simulink model "SWC_HALOUT_type"  (R2021b)
settings: Solver=FixedStepDiscrete  StartTime=0.0  StopTime=10.0  FixedStep=0.005  RelTol=1e-3
values from neighbouring files (symbols this model uses):
  DTC_10020B = Simulink.Parameter    [DTC_Constant_Definition.m]
  DTC_10020C = Simulink.Parameter    [DTC_Constant_Definition.m]
  DTC_10020D = Simulink.Parameter    [DTC_Constant_Definition.m]
  DTC_10020E = Simulink.Parameter    [DTC_Constant_Definition.m]
  DTC_100210 = Simulink.Parameter    [DTC_Constant_Definition.m]
  DTC_100211 = Simulink.Parameter    [DTC_Constant_Definition.m]
  DTC_100212 = Simulink.Parameter    [DTC_Constant_Definition.m]
  DTC_100213 = Simulink.Parameter    [DTC_Constant_Definition.m]
  DTC_100214 = Simulink.Parameter    [DTC_Constant_Definition.m]
  DTC_100215 = Simulink.Parameter    [DTC_Constant_Definition.m]
  DTC_100216 = Simulink.Parameter    [DTC_Constant_Definition.m]
  DTC_100217 = Simulink.Parameter    [DTC_Constant_Definition.m]
  DTC_100218 = Simulink.Parameter    [DTC_Constant_Definition.m]
  DTC_100219 = Simulink.Parameter    [DTC_Constant_Definition.m]
  DTC_10021A = Simulink.Parameter    [DTC_Constant_Definition.m]
  DTC_10021B = Simulink.Parameter    [DTC_Constant_Definition.m]
  DTC_10021C = Simulink.Parameter    [DTC_Constant_Definition.m]
  DTC_10021D = Simulink.Parameter    [DTC_Constant_Definition.m]
  DTC_10021E = Simulink.Parameter    [DTC_Constant_Definition.m]
  DTC_100220 = Simulink.Parameter    [DTC_Constant_Definition.m]
  DTC_100221 = Simulink.Parameter    [DTC_Constant_Definition.m]
  DTC_100223 = Simulink.Parameter    [DTC_Constant_Definition.m]
  DTC_100224 = Simulink.Parameter    [DTC_Constant_Definition.m]
  DTC_100225 = Simulink.Parameter    [DTC_Constant_Definition.m]
  DTC_100226 = Simulink.Parameter    [DTC_Constant_Definition.m]
  DTC_100227 = Simulink.Parameter    [DTC_Constant_Definition.m]
  DTC_100242 = Simulink.Parameter    [DTC_Constant_Definition.m]
  DTC_100243 = Simulink.Parameter    [DTC_Constant_Definition.m]
  DTC_100244 = Simulink.Parameter    [DTC_Constant_Definition.m]
  DTC_100247 = Simulink.Parameter    [DTC_Constant_Definition.m]
  DTC_100248 = Simulink.Parameter    [DTC_Constant_Definition.m]
  DTC_100249 = Simulink.Parameter    [DTC_Constant_Definition.m]
  DTC_100250 = Simulink.Parameter    [DTC_Constant_Definition.m]
  DTC_100251 = Simulink.Parameter    [DTC_Constant_Definition.m]
  DTC_100252 = Simulink.Parameter    [DTC_Constant_Definition.m]
  DTC_100A10 = Simulink.Parameter    [DTC_Constant_Definition.m]
  DTC_100A12 = Simulink.Parameter    [DTC_Constant_Definition.m]
  DTC_100A16 = Simulink.Parameter    [DTC_Constant_Definition.m]
  DTC_100A17 = Simulink.Parameter    [DTC_Constant_Definition.m]
  DTC_100A18 = Simulink.Parameter    [DTC_Constant_Definition.m]
  DTC_100A19 = Simulink.Parameter    [DTC_Constant_Definition.m]
  DTC_500B01 = Simulink.Parameter    [DTC_Constant_Definition.m]
  DTC_500B02 = Simulink.Parameter    [DTC_Constant_Definition.m]
  DTC_500B03 = Simulink.Parameter    [DTC_Constant_Definition.m]
  DTC_500B04 = Simulink.Parameter    [DTC_Constant_Definition.m]
  DTC_500B05 = Simulink.Parameter    [DTC_Constant_Definition.m]
  DTC_500B06 = Simulink.Parameter    [DTC_Constant_Definition.m]
  DTC_500B07 = Simulink.Parameter    [DTC_Constant_Definition.m]
  DTC_500B08 = Simulink.Parameter    [DTC_Constant_Definition.m]
  DTC_500B09 = Simulink.Parameter    [DTC_Constant_Definition.m]
  DTC_500B0A = Simulink.Parameter    [DTC_Constant_Definition.m]
  DTC_500B0B = Simulink.Parameter    [DTC_Constant_Definition.m]
  DTC_500B0C = Simulink.Parameter    [DTC_Constant_Definition.m]
  DTC_500B0D = Simulink.Parameter    [DTC_Constant_Definition.m]
  DTC_500B0E = Simulink.Parameter    [DTC_Constant_Definition.m]
  DTC_500B0F = Simulink.Parameter    [DTC_Constant_Definition.m]
  DTC_500B10 = Simulink.Parameter    [DTC_Constant_Definition.m]
  DTC_90021F = Simulink.Parameter    [DTC_Constant_Definition.m]
  DTC_90022F = Simulink.Parameter    [DTC_Constant_Definition.m]
  DTC_900253 = Simulink.Parameter    [DTC_Constant_Definition.m]
  DTC_900254 = Simulink.Parameter    [DTC_Constant_Definition.m]
  DTC_900301 = Simulink.Parameter    [DTC_Constant_Definition.m]
  DTC_900302 = Simulink.Parameter    [DTC_Constant_Definition.m]
  DTC_900303 = Simulink.Parameter    [DTC_Constant_Definition.m]
  DTC_900304 = Simulink.Parameter    [DTC_Constant_Definition.m]
  DTC_900305 = Simulink.Parameter    [DTC_Constant_Definition.m]
  DTC_900909 = Simulink.Parameter    [DTC_Constant_Definition.m]
  DTC_90090A = Simulink.Parameter    [DTC_Constant_Definition.m]
  DTC_90090B = Simulink.Parameter    [DTC_Constant_Definition.m]
  DTC_90090C = Simulink.Parameter    [DTC_Constant_Definition.m]
  DTC_90090D = Simulink.Parameter    [DTC_Constant_Definition.m]
  DTC_90090E = Simulink.Parameter    [DTC_Constant_Definition.m]
  DTC_90090F = Simulink.Parameter    [DTC_Constant_Definition.m]
  DTC_900910 = Simulink.Parameter    [DTC_Constant_Definition.m]
  DTC_900911 = Simulink.Parameter    [DTC_Constant_Definition.m]
  DTC_900912 = Simulink.Parameter    [DTC_Constant_Definition.m]
  DTC_900913 = Simulink.Parameter    [DTC_Constant_Definition.m]
  DTC_900914 = Simulink.Parameter    [DTC_Constant_Definition.m]
  DTC_C0288F = Simulink.Parameter    [DTC_Constant_Definition.m]
  DTC_C0378F = Simulink.Parameter    [DTC_Constant_Definition.m]
  DTC_C0468F = Simulink.Parameter    [DTC_Constant_Definition.m]
  DTC_C0558F = Simulink.Parameter    [DTC_Constant_Definition.m]
  DTC_C0648F = Simulink.Parameter    [DTC_Constant_Definition.m]
  DTC_C0808F = Simulink.Parameter    [DTC_Constant_Definition.m]
  DTC_D00201 = Simulink.Parameter    [DTC_Constant_Definition.m]
  DTC_D00202 = Simulink.Parameter    [DTC_Constant_Definition.m]
  DTC_D00203 = Simulink.Parameter    [DTC_Constant_Definition.m]
  DTC_D00204 = Simulink.Parameter    [DTC_Constant_Definition.m]
  DTC_D00205 = Simulink.Parameter    [DTC_Constant_Definition.m]
  DTC_D00206 = Simulink.Parameter    [DTC_Constant_Definition.m]
  DTC_D00207 = Simulink.Parameter    [DTC_Constant_Definition.m]
  DTC_D00208 = Simulink.Parameter    [DTC_Constant_Definition.m]
  DTC_D00209 = Simulink.Parameter    [DTC_Constant_Definition.m]
  DTC_D0020A = Simulink.Parameter    [DTC_Constant_Definition.m]
  DTC_D00228 = Simulink.Parameter    [DTC_Constant_Definition.m]
  DTC_D00229 = Simulink.Parameter    [DTC_Constant_Definition.m]
  DTC_D0022A = Simulink.Parameter    [DTC_Constant_Definition.m]
  DTC_D0022B = Simulink.Parameter    [DTC_Constant_Definition.m]
  DTC_D0022C = Simulink.Parameter    [DTC_Constant_Definition.m]
  DTC_D0022D = Simulink.Parameter    [DTC_Constant_Definition.m]
  DTC_D00230 = Simulink.Parameter    [DTC_Constant_Definition.m]
  DTC_D00231 = Simulink.Parameter    [DTC_Constant_Definition.m]
  DTC_D00232 = Simulink.Parameter    [DTC_Constant_Definition.m]
  DTC_D00234 = Simulink.Parameter    [DTC_Constant_Definition.m]
  DTC_D00235 = Simulink.Parameter    [DTC_Constant_Definition.m]
  DTC_D00236 = Simulink.Parameter    [DTC_Constant_Definition.m]
  DTC_D00237 = Simulink.Parameter    [DTC_Constant_Definition.m]
  DTC_D00238 = Simulink.Parameter    [DTC_Constant_Definition.m]
  DTC_D0023A = Simulink.Parameter    [DTC_Constant_Definition.m]
  DTC_D0023B = Simulink.Parameter    [DTC_Constant_Definition.m]
  DTC_D0023C = Simulink.Parameter    [DTC_Constant_Definition.m]
  DTC_D0023D = Simulink.Parameter    [DTC_Constant_Definition.m]
  DTC_D0023E = Simulink.Parameter    [DTC_Constant_Definition.m]
  DTC_D00240 = Simulink.Parameter    [DTC_Constant_Definition.m]
  DTC_D00241 = Simulink.Parameter    [DTC_Constant_Definition.m]
undefined symbols (not defined in the file or in its folder): DIDLen_APPD, DIDLen_APPE, DIDLen_APPPedalZP, DIDLen_APSFunConfig, DIDLen_AutoLock, DIDLen_AutoWipHSpdEN, DIDLen_CALID, DIDLen_CDEODT, DIDLen_CLRDIST, DIDLen_DKCBLESta, DIDLen_DKCKey, DIDLen_DKCSta, DIDLen_DoorNFCAnchorSta, DIDLen_DRLDis, DIDLen_DynoMode, DIDLen_ECUNAME, DIDLen_FDDKCCoordXY, DIDLen_FMHTimer, DIDLen_LFLowPresThre, DIDLen_LFSensorID, DIDLen_LIDAAnchorSta, DIDLen_LRLowPresThre, DIDLen_LRSensorID, DIDLen_MILDIST, DIDLen_NUMPSATRIPSFLTMEMCLR, DIDLen_NVMPedalZP, DIDLen_OBDReq, DIDLen_ODOMETER, DIDLen_PKE, DIDLen_ProtocolId, DIDLen_PSA, DIDLen_QTYPSATRIPS, DIDLen_RFLowPresThre, DIDLen_RFSensorID, DIDLen_RRLowPresThre, DIDLen_RRSensorID, DIDLen_RUNTM, DIDLen_SensorMode, DIDLen_TestGroup, DIDLen_TireSize, DIDLen_TPMSLearnSta, DIDLen_UIDSta, DIDLen_USSConfig, DIDLen_UWBAnchorSta, DIDLen_VIN, DIDLen_VSS, DIDLen_WhlPres, DIDLen_WhlSensorBattSta, DIDLen_WhlTmp, DIDLen_WipRLSCmdCutFilter, DIDLen_WipRLSCmdHoldFilter, DIDLen_XWDMode, DIDNum_APPD, DIDNum_APPE, DIDNum_APPPedalZP, DIDNum_APSFunConfig, DIDNum_AutoLock, DIDNum_AutoWipHSpdEN, DIDNum_CALID, DIDNum_CDEODT ... (+281)
libraries: simulink x213, FVT_lib x160, hdlsllib x6, hcu_lib x5, halout x1
(part 4 of 9)

== system SWC_HALOUT_type/run_SWC_HALOUT_Tx_5ms_sys/HALOUT_AFTER/R_E2E_CAN3_VCU1_CSOP_Write_CAN3_VCU1 ==
  Enable : EnablePort
  R_E2E_CAN3_VCU1_CSOP_Write_CAN3_VCU1 : FunctionCaller  FunctionPrototype=R_E2E_CAN3_VCU1_CSOP_Write_CAN3_VCU1()

== system SWC_HALOUT_type/run_SWC_HALOUT_Tx_5ms_sys/HALOUT_AFTER/R_E2E_CAN3_VCU1_toNIDEC_CSOP_Write_CAN3_VCU1_toNIDEC ==
  In1 : EnablePort
  R_E2E_CAN3_VCU1_toNIDEC_CSOP_Write_CAN3_VCU1_toNIDEC : FunctionCaller  FunctionPrototype=R_E2E_CAN3_VCU1_toNIDEC_CSOP_Write_CAN3_VCU1_toNIDEC()

== system SWC_HALOUT_type/run_SWC_HALOUT_Tx_5ms_sys/HALOUT_AFTER/R_E2E_CAN4_VCU1_CSOP_Write_CAN4_VCU1 ==
  In1 : EnablePort
  R_E2E_CAN4_VCU1_CSOP_Write_CAN4_VCU1 : FunctionCaller  FunctionPrototype=R_E2E_CAN4_VCU1_CSOP_Write_CAN4_VCU1()

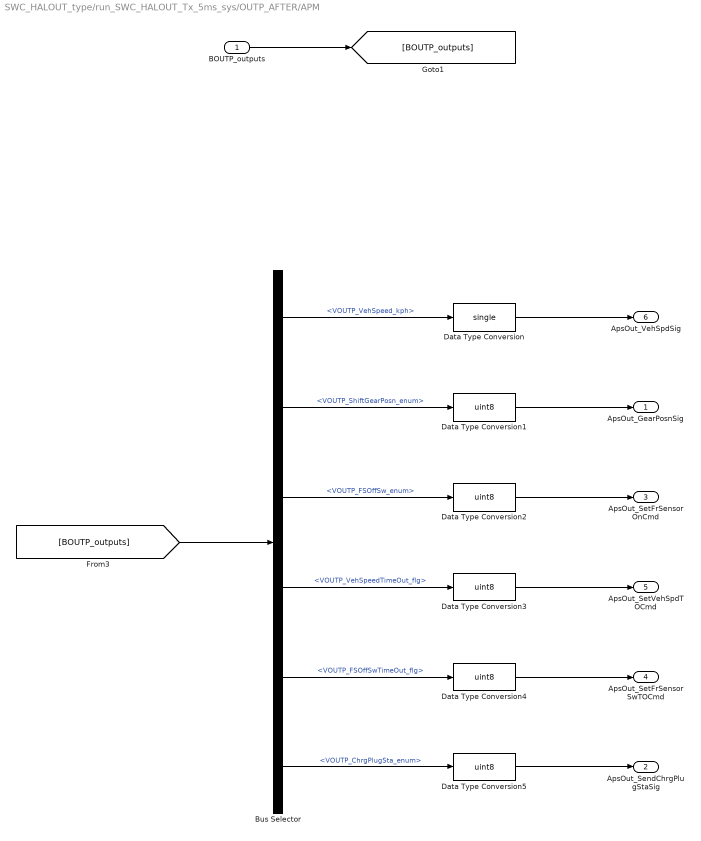
== system SWC_HALOUT_type/run_SWC_HALOUT_Tx_5ms_sys/OUTP_AFTER/APM ==
  BOUTP_outputs : Inport  OutDataTypeStr=Bus: BOUTP_outputs
  Bus Selector : BusSelector  OutputSignals=VOUTP_VehSpeed_kph,VOUTP_ShiftGearPosn_enum,VOUTP_FSOffSw_enum,VOUTP_VehSpeedTimeOut_flg,VOUTP_FSOffSwTimeOut_flg,VOUTP_ChrgPlugSta_enum
  Data Type Conversion : DataTypeConversion  OutDataTypeStr=single
  Data Type Conversion{1..5} (5 alike) : DataTypeConversion  OutDataTypeStr=uint8
  ApsOut_GearPosnSig : Outport
  ApsOut_SendChrgPlugStaSig : Outport  Port=2
  ApsOut_SetFrSensorOnCmd : Outport  Port=3
  ApsOut_SetFrSensorSwTOCmd : Outport  Port=4
  ApsOut_SetVehSpdTOCmd : Outport  Port=5
  ApsOut_VehSpdSig : Outport  Port=6
  wires:
  BOUTP_outputs/1 -> [BOUTP_outputs]
  [BOUTP_outputs] -> Bus Selector/1
  Bus Selector/1 -> Data Type Conversion/1  "<VOUTP_VehSpeed_kph>"
  Bus Selector/2 -> Data Type Conversion1/1  "<VOUTP_ShiftGearPosn_enum>"
  Bus Selector/3 -> Data Type Conversion2/1  "<VOUTP_FSOffSw_enum>"
  Bus Selector/4 -> Data Type Conversion3/1  "<VOUTP_VehSpeedTimeOut_flg>"
  Bus Selector/5 -> Data Type Conversion4/1  "<VOUTP_FSOffSwTimeOut_flg>"
  Data Type Conversion1/1 -> ApsOut_GearPosnSig/1
  Data Type Conversion2/1 -> ApsOut_SetFrSensorOnCmd/1
  Data Type Conversion4/1 -> ApsOut_SetFrSensorSwTOCmd/1
  Data Type Conversion5/1 -> ApsOut_SendChrgPlugStaSig/1
  Bus Selector/6 -> Data Type Conversion5/1  "<VOUTP_ChrgPlugSta_enum>"
  Data Type Conversion/1 -> ApsOut_VehSpdSig/1
  Data Type Conversion3/1 -> ApsOut_SetVehSpdTOCmd/1

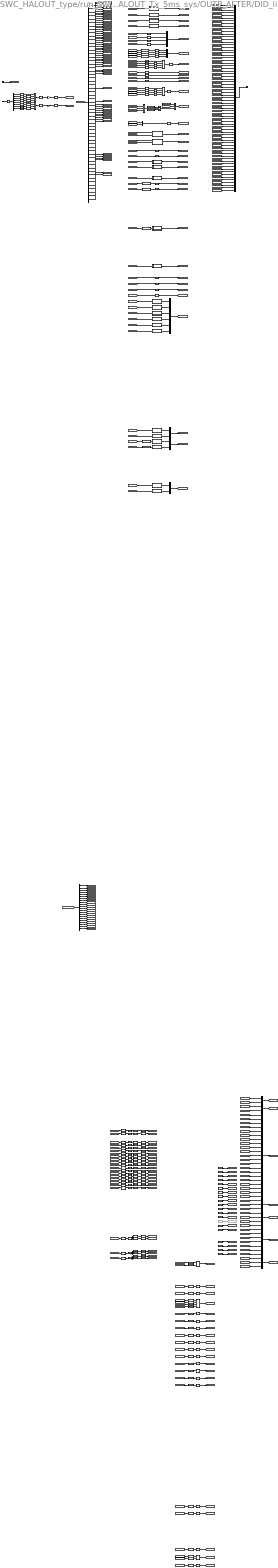
== system SWC_HALOUT_type/run_SWC_HALOUT_Tx_5ms_sys/OUTP_AFTER/DID_list ==
  BOUTP_outputs : Inport
  VHAL_NvmReadArray_raw : Inport  Port=2
  Bit Shift : hdlsllib/Logic and Bit Operations/Bit Shift  mode=Shift Left Logical  N=3
  Bit Shift1 : hdlsllib/Logic and Bit Operations/Bit Shift  mode=Shift Left Logical  N=2
  Bit Shift2 : hdlsllib/Logic and Bit Operations/Bit Shift  mode=Shift Left Logical  N=1
  Bit Shift3 : hdlsllib/Logic and Bit Operations/Bit Shift  mode=Shift Left Logical  N=3
  Bit Shift4 : hdlsllib/Logic and Bit Operations/Bit Shift  mode=Shift Left Logical  N=2
  Bit Shift5 : hdlsllib/Logic and Bit Operations/Bit Shift  mode=Shift Left Logical  N=1
  Bitwise OR : simulink/Logic and Bit Operations/Bitwise Operator  logicop=OR  UseBitMask=off  NumInputPorts=4  BitMask=bin2dec('11011001')  BitMaskRealWorld=Stored Integer
  Bitwise OR1 : simulink/Logic and Bit Operations/Bitwise Operator  logicop=OR  UseBitMask=off  NumInputPorts=4  BitMask=bin2dec('11011001')  BitMaskRealWorld=Stored Integer
  Bitwise OR13 : simulink/Logic and Bit Operations/Bitwise Operator  logicop=OR  UseBitMask=off  NumInputPorts=4  BitMask=bin2dec('00000000000000000000')  BitMaskRealWorld=Stored Integer
  Bitwise OR14 : simulink/Logic and Bit Operations/Bitwise Operator  logicop=OR  UseBitMask=off  NumInputPorts=4  BitMask=bin2dec('00000000000000000000')  BitMaskRealWorld=Stored Integer
  BitwiseAND{40..41,44..60,63..64,69..72} (25 alike) : simulink/Logic and Bit Operations/Bitwise Operator  logicop=AND  UseBitMask=on  BitMask=0xFF  BitMaskRealWorld=Stored Integer
  BitwiseOR53 : simulink/Logic and Bit Operations/Bitwise Operator  logicop=OR  UseBitMask=off  NumInputPorts=2  BitMask=bin2dec('11011001')  BitMaskRealWorld=Stored Integer
  BitwiseOR{56..57,59..69,86..87,92,94} (17 alike) : simulink/Logic and Bit Operations/Bitwise Operator  logicop=OR  UseBitMask=off  BitMask=bin2dec('11011001')  BitMaskRealWorld=Stored Integer
  BitwiseOR58 : simulink/Logic and Bit Operations/Bitwise Operator  logicop=OR  UseBitMask=off  NumInputPorts=4  BitMask=bin2dec('11011001')  BitMaskRealWorld=Stored Integer
  BitwiseOR93 : simulink/Logic and Bit Operations/Bitwise Operator  logicop=OR  UseBitMask=off  NumInputPorts=2  BitMask=bin2dec('11011001')  BitMaskRealWorld=Stored Integer
  Bus Creator : BusCreator  Inputs=71
  Bus Selector : BusSelector  OutputSignals=VOUTP_WriteChkLFID_raw,VOUTP_WriteChkRFID_raw,VOUTP_WriteChkLRID_raw,VOUTP_WriteChkRRID_raw,VOUTP_LFWheelPress_raw8,VOUTP_RFWheelPress_raw8,VOUTP_LRWheelPress_raw8,VOUTP_RRWheelPress_raw8,VOUTP_LFWheelTemp_C,VOUTP_RFWheelTemp_C,VOUTP_LRWheelTemp_C,VOUTP_RRWheelTemp_C,VOUTP_LFBatWarn_flg,VOUTP_RFBatWarn_flg,VOUTP_LRBatWarn_flg,VOUTP_RRBatWarn_flg,VOUTP_LFWheelPSW_raw8,VOUTP_LRWheelPSW_raw8,VOUTP_RFWheelPSW_raw8,VOUTP_RRWheelPSW_raw8,VOUTP_LFSensorMode_flg,VOUTP_RFSensorMode_flg,VOUTP_LRSensorMode_flg,VOUTP_RRSensorMode_flg,VOUTP_ALFin_flg,VOUTP_ChkStorge_flg,VOUTP_TPMSStorge_flg,VOUTP_unlearnSfali_flg,VOUTP_WritingCnt_enum,VOUTP_LProgress_enum,VOUTP_EAPS1MIN_pct,VOUTP_EAPS2MIN_pct,VOUTP_DrivetrainSelect_enum,VOUTP_VSS_kph,VOUTP_RUNTM_s,VOUTP_MILDIST_km,VOUTP_CLRDIST_km,VOUTP_APPD_pct,VOUTP_APPE_pct,VOUTP_ODOMETER_km,VOUTP_NUMPSATRIPSFLTMEMCLR_cnt,VOUTP_VinCode_cnt,VOUTP_CALID_cnt,VOUTP_ECUNAME_cnt,VOUTP_PROTOCOLID_enum,VOUTP_PSAR_sec,VOUTP_PSAL_sec,VOUTP_IPSAR_sec,VOUTP_IPSAL_sec,VOUTP_CPSAR_sec,VOUTP_CPSAL_sec,VOUTP_PKER_kphsqr,VOUTP_PKEL_kphsqr,VOUTP_CDEODTR_km,VOUTP_CDEODTL_km,VOUTP_QTYPSATRIPSR_cnt,VOUTP_QTYPSATRIPSL_cnt
  Constant : Constant  Value=ENUM_TPMSLearnStatus_LEARNFAIL
  Constant1 : Constant  Value=ENUM_TPMSLearnStatus_NOTLEARN
  Constant{3..10,12..13,15..18} (14 alike) : Constant  Value=zeros(10,1)  OutDataTypeStr=uint8
  Constant{11,19,21..23} (5 alike) : Constant  Value=zeros(1,1)  OutDataTypeStr=uint8
  Constant14 : Constant  Commented=on  Value=zeros(1,1)  OutDataTypeStr=uint8
  Constant2 : Constant  Value=ENUM_TPMSLearnStatus_LEARNED
  Data Type Conversion{1..25,27,29,33..36,94..95,98..100,102..111,113..116,135..136,141..144} (56 alike) : DataTypeConversion  OutDataTypeStr=uint8
  Data Type Conversion168 : DataTypeConversion  OutDataTypeStr=single
  Data Type Conversion{169..178} (10 alike) : DataTypeConversion  OutDataTypeStr=uint32
  Data Type Conversion179 : DataTypeConversion  OutDataTypeStr=single
  Demux : Demux  Outputs=8
  Goto191 : Goto  Commented=on  GotoTag=DoorNFCanchorStatus3
  LeftShift40 : ArithShift  BitShiftNumber=4  BitShiftDirection=Left
  LeftShift{41,44..45,49..60} (15 alike) : ArithShift  BitShiftDirection=Left
  LeftShift46 : ArithShift  BitShiftNumber=6  BitShiftDirection=Left
  LeftShift47 : ArithShift  BitShiftNumber=4  BitShiftDirection=Left
  LeftShift48 : ArithShift  BitShiftNumber=2  BitShiftDirection=Left
  Logical Operator1 : Logic  Operator=OR  Inputs=3  AllPortsSameDT=off  OutDataTypeStr=boolean
  Multiply1 : Gain  Gain=1/10000
  Multiply2 : Gain  Gain=1/10000
  Mux : Mux
  Mux{1,14..15,19,31..32} (6 alike) : Mux  Inputs=2
  Mux2 : Mux
  Mux33 : Mux  Inputs=21
  Mux34 : Mux  Inputs=3
  Mux35 : Mux  Inputs=3
  Mux36 : Mux  Inputs=8
  Mux37 : Mux  Inputs=3
  Mux6 : Mux  Inputs=6
  RightShift : ArithShift  BitShiftNumber=8
  RightShift1 : ArithShift
  RightShift6 : ArithShift  BitShiftNumber=1
  RightShift7 : ArithShift  BitShiftNumber=-7
  RightShift8 : ArithShift  BitShiftNumber=2
  RightShift9 : ArithShift  BitShiftNumber=-6
  Selector1 : Selector  InputPortWidth=1024  IndexOptions=Index vector (dialog)  Indices=[112:119]  OutputSizes=1
  Shift Arithmetic37 : ArithShift  BitShiftNumber=8  BitShiftDirection=Left
  Shift Arithmetic38 : ArithShift  BitShiftNumber=16  BitShiftDirection=Left
  Shift Arithmetic39 : ArithShift  BitShiftNumber=24  BitShiftDirection=Left
  Shift Arithmetic40 : ArithShift  BitShiftNumber=8  BitShiftDirection=Left
  Shift Arithmetic41 : ArithShift  BitShiftNumber=16  BitShiftDirection=Left
  Shift Arithmetic42 : ArithShift  BitShiftNumber=24  BitShiftDirection=Left
  Switch : Switch  Criteria=u2 ~= 0
  Switch1 : Switch  Criteria=u2 ~= 0
  UnitConverter{56..57,60..76} (19 alike) : DataTypeConversion  OutDataTypeStr=uint8
  UnitConverter93 : DataTypeConversion  OutDataTypeStr=uint16
  UnitConverter96 : DataTypeConversion  OutDataTypeStr=uint16
  UnitConverter97 : DataTypeConversion  OutDataTypeStr=uint16
  bus_selector : BusSelector  OutputSignals=VOUTP_KeyModeSta_enum,VOUTP_UWBDetArea_enum,VOUTP_BLERSSI_enum,VOUTP_UWBOnOff_flg,VOUTP_UWB1Invalid_flg,VOUTP_UWB2Invalid_flg,VOUTP_UWB3Invalid_flg,VOUTP_UWB4Invalid_flg,VOUTP_UWB0Invalid_flg,VOUTP_UWB1FPP_enum,VOUTP_UWB2FPP_enum,VOUTP_UWB3FPP_enum,VOUTP_UWB4FPP_enum,VOUTP_UWB0FPP_enum,VOUTP_UWB1Distance_enum,VOUTP_UWB2Distance_enum,VOUTP_UWB3Distance_enum,VOUTP_UWB4Distance_enum,VOUTP_UWB0Distance_enum,VOUTP_UIDBatVolt_enum,VOUTP_CoordinateX_enum,VOUTP_CoordinateY_enum
  convert_in : FVT_lib/hal/convert_in  gain=10  offset=0
  convert_in12 : FVT_lib/hal/convert_in  gain=10  offset=0
  convert_in13 : FVT_lib/hal/convert_in  gain=10  offset=0
  convert_in28 : FVT_lib/hal/convert_in  gain=2.55  offset=0
  convert_in29 : FVT_lib/hal/convert_in  gain=2.55  offset=0
  convert_out{,1..3} (4 alike) : FVT_lib/hal/convert_out  gain=1  offset=-40
  convert_out100 : FVT_lib/hal/convert_out  gain=10  offset=-2550
  convert_out101 : FVT_lib/hal/convert_out  gain=10  offset=-2550
  convert_out{56..57,61..67} (9 alike) : FVT_lib/hal/convert_out  gain=1  offset=0
  convert_out{68..70,72..73} (5 alike) : FVT_lib/hal/convert_out  gain=1  offset=-127
  convert_out{74..78,97} (6 alike) : FVT_lib/hal/convert_out  gain=10  offset=0
  pct2raw1 : Subsystem
  pct2raw8 : Subsystem
  uint16Touint8Array1 : Subsystem
  uint16Touint8Array12 : Subsystem
  uint16Touint8Array2 : Subsystem
  uint16Touint8Array3 : Subsystem
  uint32Touint8Array : Subsystem
  uint32Touint8Array1 : Subsystem
  uint32Touint8Array10 : Subsystem
  uint32Touint8Array11 : Subsystem
  uint32Touint8Array12 : Subsystem
  uint32Touint8Array2 : Subsystem
  uint32Touint8Array29 : Subsystem
  uint32Touint8Array3 : Subsystem
  uint32Touint8Array30 : Subsystem
  uint32Touint8Array31 : Subsystem
  uint32Touint8Array32 : Subsystem
  uint32Touint8Array33 : Subsystem
  uint32Touint8Array34 : Subsystem
  uint32Touint8Array4 : Subsystem
  uint32Touint8Array7 : Subsystem
  uint32Touint8Array8 : Subsystem
  uint32Touint8Array9 : Subsystem
  BOUTP_DIDSetData_outputs : Outport
  wires:
  Bus Selector/1 -> [VOUTP_WriteChkLFID_raw]  "<VOUTP_WriteChkLFID_raw>"
  Bus Selector/2 -> [VOUTP_WriteChkRFID_raw]  "<VOUTP_WriteChkRFID_raw>"
  Bus Selector/4 -> [VOUTP_WriteChkRRID_raw]  "<VOUTP_WriteChkRRID_raw>"
  Bus Selector/3 -> [VOUTP_WriteChkLRID_raw]  "<VOUTP_WriteChkLRID_raw>"
  Bus Selector/5 -> [VOUTP_LFWheelPress_raw8]  "<VOUTP_LFWheelPress_raw8>"
  Bus Selector/6 -> [VOUTP_RFWheelPress_raw8]  "<VOUTP_RFWheelPress_raw8>"
  Bus Selector/7 -> [VOUTP_LRWheelPress_raw8]  "<VOUTP_LRWheelPress_raw8>"
  Bus Selector/8 -> [VOUTP_RRWheelPress_raw8]  "<VOUTP_RRWheelPress_raw8>"
  Bus Selector/13 -> [VOUTP_LFBatWarn_flg]  "<VOUTP_LFBatWarn_flg>"
  Bus Selector/14 -> [VOUTP_RFBatWarn_flg]  "<VOUTP_RFBatWarn_flg>"
  Bus Selector/15 -> [VOUTP_LRBatWarn_flg]  "<VOUTP_LRBatWarn_flg>"
  Bus Selector/16 -> [VOUTP_RRBatWarn_flg]  "<VOUTP_RRBatWarn_flg>"
  Bus Selector/18 -> [VOUTP_LRWheelPSW_raw8]  "<VOUTP_LRWheelPSW_raw8>"
  Bus Selector/19 -> [VOUTP_RFWheelPSW_raw8]  "<VOUTP_RFWheelPSW_raw8>"
  Bus Selector/20 -> [VOUTP_RRWheelPSW_raw8]  "<VOUTP_RRWheelPSW_raw8>"
  Bus Selector/17 -> [VOUTP_LFWheelPSW_raw8]  "<VOUTP_LFWheelPSW_raw8>"
  Bus Selector/21 -> [VOUTP_LFSensorMode_flg]  "<VOUTP_LFSensorMode_flg>"
  Bus Selector/22 -> [VOUTP_RFSensorMode_flg]  "<VOUTP_RFSensorMode_flg>"
  Bus Selector/23 -> [VOUTP_LRSensorMode_flg]  "<VOUTP_LRSensorMode_flg>"
  Bus Selector/24 -> [VOUTP_RRSensorMode_flg]  "<VOUTP_RRSensorMode_flg>"
  Bus Selector/27 -> [VOUTP_TPMSStorge_flg]  "<VOUTP_TPMSStorge_flg>"
  Bus Selector/25 -> [VOUTP_ALFin_flg]  "<VOUTP_ALFin_flg>"
  Bus Selector/26 -> [VOUTP_ChkStorge_flg]  "<VOUTP_ChkStorge_flg>"
  Bus Selector/28 -> [VOUTP_unlearnSfali_flg]  "<VOUTP_unlearnSfali_flg>"
  Bus Selector/9 -> [VOUTP_LFWheelTemp_C]  "<VOUTP_LFWheelTemp_C>"
  Bus Selector/10 -> [VOUTP_RFWheelTemp_C]  "<VOUTP_RFWheelTemp_C>"
  Bus Selector/11 -> [VOUTP_LRWheelTemp_C]  "<VOUTP_LRWheelTemp_C>"
  Bus Selector/12 -> [VOUTP_RRWheelTemp_C]  "<VOUTP_RRWheelTemp_C>"
  Data Type Conversion8/1 -> Mux2/1
  Data Type Conversion9/1 -> Mux2/2
  Data Type Conversion10/1 -> Mux2/3
  Data Type Conversion11/1 -> Mux2/4
  [VOUTP_LFWheelPSW_raw8] -> Data Type Conversion6/1
  [VOUTP_RRWheelPSW_raw8] -> Data Type Conversion5/1
  [VOUTP_LFSensorMode_flg] -> Data Type Conversion21/1
  [VOUTP_RRSensorMode_flg] -> Data Type Conversion14/1
  [VOUTP_LRSensorMode_flg] -> Data Type Conversion12/1
  [VOUTP_RFSensorMode_flg] -> Data Type Conversion13/1
  Data Type Conversion21/1 -> Bitwise OR/1
  Data Type Conversion12/1 -> Bit Shift1/1
  Data Type Conversion14/1 -> Bit Shift/1
  Constant1/1 -> Switch1/3
  [VOUTP_ALFin_flg] -> Logical Operator1/1
  Switch1/1 -> Switch/3
  [VOUTP_ChkStorge_flg] -> Logical Operator1/2
  Constant/1 -> Switch/1
  Constant2/1 -> Switch1/1
  [VOUTP_TPMSStorge_flg] -> Logical Operator1/3
  Logical Operator1/1 -> Switch1/2
  [VOUTP_unlearnSfali_flg] -> Switch/2
  Mux/1 -> [VHAL_DIDSetWhlPres_raw8]
  Mux2/1 -> [VHAL_DIDSetWhlTmp_raw8]
  Data Type Conversion6/1 -> [VHAL_DIDSetLFLowPresThre_raw8]
  Data Type Conversion7/1 -> [VHAL_DIDSetRFLowPresThre_raw8]
  Data Type Conversion4/1 -> [VHAL_DIDSetLRLowPresThre_raw8]
  Data Type Conversion5/1 -> [VHAL_DIDSetRRLowPresThre_raw8]
  Bitwise OR/1 -> Data Type Conversion20/1
  Switch/1 -> [VHAL_DIDSetTPMSLearnSta_raw8]
  Bit Shift/1 -> Bitwise OR/4
  Bit Shift1/1 -> Bitwise OR/3
  Bit Shift2/1 -> Bitwise OR/2
  Data Type Conversion20/1 -> [VHAL_DIDSetSensorMode_raw8]
  Data Type Conversion13/1 -> Bit Shift2/1
  [VOUTP_RFBatWarn_flg] -> Data Type Conversion2/1
  Data Type Conversion1/1 -> Bit Shift4/1
  [VOUTP_LRBatWarn_flg] -> Data Type Conversion1/1
  [VOUTP_LFBatWarn_flg] -> Data Type Conversion22/1
  Bitwise OR1/1 -> Data Type Conversion15/1
  Bit Shift4/1 -> Bitwise OR1/3
  Data Type Conversion2/1 -> Bit Shift5/1
  Bit Shift3/1 -> Bitwise OR1/4
  Data Type Conversion22/1 -> Bitwise OR1/1
  Data Type Conversion3/1 -> Bit Shift3/1
  Bit Shift5/1 -> Bitwise OR1/2
  [VOUTP_RRBatWarn_flg] -> Data Type Conversion3/1
  Data Type Conversion15/1 -> [VHAL_DIDSetWhlSensorBattSta_raw8]
  [VHAL_DIDSetTPMSLearnSta_raw8] -> Bus Creator/13  "VHAL_DIDSetTPMSLearnSta_raw8"
  [VHAL_DIDSetLFSensorID_raw8] -> Bus Creator/1  "VHAL_DIDSetLFSensorID_raw8"
  [VHAL_DIDSetRFSensorID_raw8] -> Bus Creator/2  "VHAL_DIDSetRFSensorID_raw8"
  [VHAL_DIDSetLRSensorID_raw8] -> Bus Creator/3  "VHAL_DIDSetLRSensorID_raw8"
  [VHAL_DIDSetRRSensorID_raw8] -> Bus Creator/4  "VHAL_DIDSetRRSensorID_raw8"
  [VHAL_DIDSetWhlPres_raw8] -> Bus Creator/5  "VHAL_DIDSetWhlPres_raw8"
  [VHAL_DIDSetWhlTmp_raw8] -> Bus Creator/6  "VHAL_DIDSetWhlTmp_raw8"
  [VHAL_DIDSetWhlSensorBattSta_raw8] -> Bus Creator/7  "VHAL_DIDSetWhlSensorBattSta_raw8"
  [VHAL_DIDSetLFLowPresThre_raw8] -> Bus Creator/8  "VHAL_DIDSetLFLowPresThre_raw8"
  [VHAL_DIDSetRFLowPresThre_raw8] -> Bus Creator/9  "VHAL_DIDSetRFLowPresThre_raw8"
  [VHAL_DIDSetLRLowPresThre_raw8] -> Bus Creator/10  "VHAL_DIDSetLRLowPresThre_raw8"
  [VHAL_DIDSetRRLowPresThre_raw8] -> Bus Creator/11  "VHAL_DIDSetRRLowPresThre_raw8"
  [VHAL_DIDSetSensorMode_raw8] -> Bus Creator/12  "VHAL_DIDSetSensorMode_raw8"
  Bus Creator/1 -> BOUTP_DIDSetData_outputs/1
  [VOUTP_WriteChkLFID_raw] -> uint32Touint8Array/1(In1)
  uint32Touint8Array/1(Out1) -> [VHAL_DIDSetLFSensorID_raw8]
  [VOUTP_WriteChkRFID_raw] -> uint32Touint8Array1/1(In1)
  uint32Touint8Array1/1(Out1) -> [VHAL_DIDSetRFSensorID_raw8]
  [VOUTP_WriteChkLRID_raw] -> uint32Touint8Array2/1(In1)
  uint32Touint8Array2/1(Out1) -> [VHAL_DIDSetLRSensorID_raw8]
  [VOUTP_WriteChkRRID_raw] -> uint32Touint8Array3/1(In1)
  uint32Touint8Array3/1(Out1) -> [VHAL_DIDSetRRSensorID_raw8]
  [VOUTP_RFWheelPress_raw8] -> Data Type Conversion17/1
  [VOUTP_LFWheelPress_raw8] -> Data Type Conversion16/1
  [VOUTP_LRWheelPress_raw8] -> Data Type Conversion18/1
  [VOUTP_RRWheelPress_raw8] -> Data Type Conversion19/1
  convert_out/1 -> Data Type Conversion8/1
  convert_out1/1 -> Data Type Conversion9/1
  convert_out2/1 -> Data Type Conversion10/1
  convert_out3/1 -> Data Type Conversion11/1
  Data Type Conversion16/1 -> Mux/1
  Data Type Conversion17/1 -> Mux/2
  Data Type Conversion18/1 -> Mux/3
  Data Type Conversion19/1 -> Mux/4
  [VOUTP_LFWheelTemp_C] -> convert_out/1
  [VOUTP_RFWheelTemp_C] -> convert_out1/1
  [VOUTP_LRWheelTemp_C] -> convert_out2/1
  [VOUTP_RRWheelTemp_C] -> convert_out3/1
  [VOUTP_RFWheelPSW_raw8] -> Data Type Conversion7/1
  [VOUTP_LRWheelPSW_raw8] -> Data Type Conversion4/1
  Bus Selector/29 -> [VOUTP_WritingCnt_enum]  "<VOUTP_WritingCnt_enum>"
  Bus Selector/30 -> [VOUTP_LProgress_enum]  "<VOUTP_LProgress_enum>"
  [VOUTP_WritingCnt_enum] -> Mux1/2
  [VHAL_TPMSSensorIDRegResults_raw8] -> Bus Creator/14  "VHAL_TPMSSensorIDRegResults_raw8"
  Data Type Conversion23/1 -> [VHAL_TPMSSensorIDRegResults_raw8]
  [VOUTP_LProgress_enum] -> Mux1/1
  Mux1/1 -> Data Type Conversion23/1
  pct2raw8/1(PedalZP_raw8) -> [VHAL_DIDSetAPPPedalZP_raw8]
  pct2raw1/1(PedalZP_raw8) -> [VHAL_DIDSetNVMPedalZP_raw8]
  [VHAL_DIDSetAPPPedalZP_raw8] -> Bus Creator/15  "VHAL_DIDSetAPPPedalZP_raw8"
  [VHAL_DIDSetNVMPedalZP_raw8] -> Bus Creator/16  "VHAL_DIDSetNVMPedalZP_raw8"
  Data Type Conversion174/1 -> Bitwise OR14/1
  Demux/7 -> Data Type Conversion176/1
  Data Type Conversion170/1 -> Shift Arithmetic37/1
  Demux/2 -> Data Type Conversion170/1
  Data Type Conversion168/1 -> [VHAL_EAPS2MINMem_pct]
  Data Type Conversion172/1 -> Shift Arithmetic39/1
  Data Type Conversion169/1 -> Bitwise OR13/1
  Data Type Conversion175/1 -> Shift Arithmetic40/1
  Data Type Conversion176/1 -> Shift Arithmetic41/1
  Data Type Conversion173/1 -> Multiply1/1
  Data Type Conversion177/1 -> Shift Arithmetic42/1
  Data Type Conversion178/1 -> Multiply2/1
  Multiply2/1 -> Data Type Conversion168/1
  Data Type Conversion171/1 -> Shift Arithmetic38/1
  Demux/8 -> Data Type Conversion177/1
  Demux/5 -> Data Type Conversion174/1
  Demux/6 -> Data Type Conversion175/1
  Bitwise OR13/1 -> Data Type Conversion173/1
  Shift Arithmetic41/1 -> Bitwise OR14/3
  Demux/3 -> Data Type Conversion171/1
  Bitwise OR14/1 -> Data Type Conversion178/1
  Shift Arithmetic39/1 -> Bitwise OR13/4
  Multiply1/1 -> Data Type Conversion179/1
  Shift Arithmetic38/1 -> Bitwise OR13/3
  Demux/4 -> Data Type Conversion172/1
  Data Type Conversion179/1 -> [VHAL_EAPS1MINMem_pct]
  Shift Arithmetic42/1 -> Bitwise OR14/4
  Shift Arithmetic40/1 -> Bitwise OR14/2
  Shift Arithmetic37/1 -> Bitwise OR13/2
  Demux/1 -> Data Type Conversion169/1
  Selector1/1 -> Demux/1
  VHAL_NvmReadArray_raw/1 -> Selector1/1
  Bus Selector/31 -> [VOUTP_EAPS1MIN_pct]  "<VOUTP_EAPS1MIN_pct>"
  Bus Selector/32 -> [VOUTP_EAPS2MIN_pct]  "<VOUTP_EAPS2MIN_pct>"
  [VOUTP_EAPS1MIN_pct] -> pct2raw8/1(EAPS1_pct)
  [VOUTP_EAPS2MIN_pct] -> pct2raw8/2(EAPS2_pct)
  [VHAL_EAPS1MINMem_pct] -> pct2raw1/1(EAPS1_pct)
  [VHAL_EAPS2MINMem_pct] -> pct2raw1/2(EAPS2_pct)
  Bus Selector/33 -> [VOUTP_DrivetrainSelect_enum]  "<VOUTP_DrivetrainSelect_enum>"
  [VOUTP_DrivetrainSelect_enum] -> Data Type Conversion24/1
  Data Type Conversion24/1 -> [VHAL_DIDSetXWDMode_raw8]
  [VHAL_DIDSetXWDMode_raw8] -> Bus Creator/17  "VHAL_DIDSetXWDMode_raw8"
  Bus Selector/41 -> [VOUTP_NUMPSATRIPSFLTMEMCLR_cnt]  "<VOUTP_NUMPSATRIPSFLTMEMCLR_cnt>"
  Bus Selector/42 -> [VOUTP_VinCode_cnt]  "<VOUTP_VinCode_cnt>"
  Bus Selector/43 -> [VOUTP_CALID_cnt]  "<VOUTP_CALID_cnt>"
  Bus Selector/44 -> [VOUTP_ECUNAME_cnt]  "<VOUTP_ECUNAME_cnt>"
  Bus Selector/45 -> [VOUTP_PROTOCOLID_enum]  "<VOUTP_PROTOCOLID_enum>"
  Bus Selector/46 -> [VOUTP_PSAR_sec]  "<VOUTP_PSAR_sec>"
  Bus Selector/47 -> [VOUTP_PSAL_sec]  "<VOUTP_PSAL_sec>"
  Bus Selector/48 -> [VOUTP_IPSAR_sec]  "<VOUTP_IPSAR_sec>"
  Bus Selector/49 -> [VOUTP_IPSAL_sec]  "<VOUTP_IPSAL_sec>"
  Bus Selector/50 -> [VOUTP_CPSAR_sec]  "<VOUTP_CPSAR_sec>"
  Bus Selector/51 -> [VOUTP_CPSAL_sec]  "<VOUTP_CPSAL_sec>"
  Bus Selector/34 -> [VOUTP_VSS_kph]  "<VOUTP_VSS_kph>"
  Bus Selector/35 -> [VOUTP_RUNTM_s]  "<VOUTP_RUNTM_s>"
  Bus Selector/36 -> [VOUTP_MILDIST_km]  "<VOUTP_MILDIST_km>"
  Bus Selector/37 -> [VOUTP_CLRDIST_km]  "<VOUTP_CLRDIST_km>"
  Bus Selector/38 -> [VOUTP_APPD_pct]  "<VOUTP_APPD_pct>"
  Bus Selector/39 -> [VOUTP_APPE_pct]  "<VOUTP_APPE_pct>"
  Bus Selector/40 -> [VOUTP_ODOMETER_km]  "<VOUTP_ODOMETER_km>"
  Bus Selector/57 -> [VOUTP_QTYPSATRIPSL_cnt]  "<VOUTP_QTYPSATRIPSL_cnt>"
  Bus Selector/52 -> [VOUTP_PKER_kphsqr]  "<VOUTP_PKER_kphsqr>"
  Bus Selector/53 -> [VOUTP_PKEL_kphsqr]  "<VOUTP_PKEL_kphsqr>"
  Bus Selector/54 -> [VOUTP_CDEODTR_km]  "<VOUTP_CDEODTR_km>"
  Bus Selector/55 -> [VOUTP_CDEODTL_km]  "<VOUTP_CDEODTL_km>"
  Bus Selector/56 -> [VOUTP_QTYPSATRIPSR_cnt]  "<VOUTP_QTYPSATRIPSR_cnt>"
  [VOUTP_VSS_kph] -> Data Type Conversion25/1
  Data Type Conversion25/1 -> [VHAL_DIDSetVSS_raw8]
  [VOUTP_RUNTM_s] -> uint16Touint8Array2/1(In1)
  [VOUTP_MILDIST_km] -> uint16Touint8Array1/1(In1)
  [VOUTP_CLRDIST_km] -> uint16Touint8Array3/1(In1)
  [VOUTP_NUMPSATRIPSFLTMEMCLR_cnt] -> uint16Touint8Array12/1(In1)
  [VOUTP_VinCode_cnt] -> Data Type Conversion33/1
  [VOUTP_CALID_cnt] -> Data Type Conversion34/1
  [VOUTP_ECUNAME_cnt] -> Data Type Conversion35/1
  [VOUTP_PROTOCOLID_enum] -> Data Type Conversion36/1
  [VOUTP_PSAR_sec] -> uint32Touint8Array7/1(In1)
  [VOUTP_PSAL_sec] -> uint32Touint8Array8/1(In1)
  [VOUTP_IPSAR_sec] -> uint32Touint8Array9/1(In1)
  [VOUTP_IPSAL_sec] -> uint32Touint8Array10/1(In1)
  [VOUTP_CPSAR_sec] -> uint32Touint8Array12/1(In1)
  [VOUTP_CPSAL_sec] -> uint32Touint8Array11/1(In1)
  [VOUTP_PKER_kphsqr] -> uint32Touint8Array29/1(In1)
  [VOUTP_PKEL_kphsqr] -> uint32Touint8Array30/1(In1)
  convert_in12/1 -> uint32Touint8Array31/1(In1)
  convert_in13/1 -> uint32Touint8Array32/1(In1)
  [VOUTP_QTYPSATRIPSR_cnt] -> uint32Touint8Array33/1(In1)
  [VOUTP_QTYPSATRIPSL_cnt] -> uint32Touint8Array34/1(In1)
  uint16Touint8Array2/1(Out1) -> [VHAL_DIDSetRUNTM_raw8]
  uint16Touint8Array1/1(Out1) -> [VHAL_DIDSetMILDIST_raw8]
  uint16Touint8Array3/1(Out1) -> [VHAL_DIDSetCLRDIST_raw8]
  Data Type Conversion27/1 -> [VHAL_DIDSetAPPD_raw8]
  Data Type Conversion29/1 -> [VHAL_DIDSetAPPE_raw8]
  uint32Touint8Array4/1(Out1) -> [VHAL_DIDSetODOMETER_raw8]
  uint16Touint8Array12/1(Out1) -> [VHAL_DIDSetNUMPSATRIPSFLTMEMCLR_raw8]
  Data Type Conversion33/1 -> [VHAL_DIDSetVIN_raw8]
  Data Type Conversion34/1 -> [VHAL_DIDSetCALID_raw8]
  Data Type Conversion35/1 -> [VHAL_DIDSetECUNAME_raw8]
  Data Type Conversion36/1 -> [VHAL_DIDSetProtocolId_raw8]
  uint32Touint8Array7/1(Out1) -> Mux6/1
  uint32Touint8Array8/1(Out1) -> Mux6/2
  uint32Touint8Array9/1(Out1) -> Mux6/3
  uint32Touint8Array10/1(Out1) -> Mux6/4
  uint32Touint8Array12/1(Out1) -> Mux6/5
  uint32Touint8Array11/1(Out1) -> Mux6/6
  Mux6/1 -> [VHAL_DIDSetPSA_raw8]
  Mux14/1 -> [VHAL_DIDSetPKE_raw8]
  uint32Touint8Array30/1(Out1) -> Mux14/2
  uint32Touint8Array29/1(Out1) -> Mux14/1
  uint32Touint8Array31/1(Out1) -> Mux15/1
  uint32Touint8Array32/1(Out1) -> Mux15/2
  Mux15/1 -> [VHAL_DIDSetCDEODT_raw8]
  Mux19/1 -> [VHAL_DIDSetQTYPSATRIPS_raw8]
  uint32Touint8Array34/1(Out1) -> Mux19/2
  uint32Touint8Array33/1(Out1) -> Mux19/1
  [VHAL_DIDSetRUNTM_raw8] -> Bus Creator/19  "VHAL_DIDSetRUNTM_raw8"
  [VHAL_DIDSetVSS_raw8] -> Bus Creator/18  "VHAL_DIDSetVSS_raw8"
  [VHAL_DIDSetMILDIST_raw8] -> Bus Creator/20  "VHAL_DIDSetMILDIST_raw8"
  [VHAL_DIDSetCLRDIST_raw8] -> Bus Creator/22  "VHAL_DIDSetCLRDIST_raw8"
  [VHAL_DIDSetWARMUPS_raw8] -> Bus Creator/21  "VHAL_DIDSetWARMUPS_raw8"
  [VHAL_DIDSetAPPD_raw8] -> Bus Creator/23  "VHAL_DIDSetAPPD_raw8"
  [VHAL_DIDSetAPPE_raw8] -> Bus Creator/24  "VHAL_DIDSetAPPE_raw8"
  [VHAL_DIDSetMILTIME_raw8] -> Bus Creator/25  "VHAL_DIDSetMILTIME_raw8"
  [VHAL_DIDSetCLRTIME_raw8] -> Bus Creator/26  "VHAL_DIDSetCLRTIME_raw8"
  [VHAL_DIDSetBATSOC_raw8] -> Bus Creator/27  "VHAL_DIDSetBATSOC_raw8"
  [VHAL_DIDSetHEVVehSysData_raw8] -> Bus Creator/28  "VHAL_DIDSetHEVVehSysData_raw8"
  [VHAL_DIDSetODOMETER_raw8] -> Bus Creator/29  "VHAL_DIDSetODOMETER_raw8"
  [VHAL_DIDSetBATSOH_raw8] -> Bus Creator/30  "VHAL_DIDSetBATSOH_raw8"
  [VHAL_DIDSetHVBCellVoltMinMax_raw8] -> Bus Creator/31  "VHAL_DIDSetHVBCellVoltMinMax_raw8"
  [VHAL_DIDSetHVESSCHARGE_raw8] -> Bus Creator/32  "VHAL_DIDSetHVESSCHARGE_raw8"
  [VHAL_DIDSetNUMPSATRIPSFLTMEMCLR_raw8] -> Bus Creator/34  "VHAL_DIDSetNUMPSATRIPSFLTMEMCLR_raw8"
  [VHAL_DIDSetHVESSENER_raw8] -> Bus Creator/33  "VHAL_DIDSetHVESSENER_raw8"
  [VHAL_DIDSetHVBattCurr_raw8] -> Bus Creator/35  "VHAL_DIDSetHVBattCurr_raw8"
  [VHAL_DIDSetVIN_raw8] -> Bus Creator/36  "VHAL_DIDSetVIN_raw8"
  [VHAL_DIDSetCALID_raw8] -> Bus Creator/37  "VHAL_DIDSetCALID_raw8"
  [VHAL_DIDSetECUNAME_raw8] -> Bus Creator/38  "VHAL_DIDSetECUNAME_raw8"
  [VHAL_DIDSetProtocolId_raw8] -> Bus Creator/39  "VHAL_DIDSetProtocolId_raw8"
  [VHAL_DIDSetPSA_raw8] -> Bus Creator/40  "VHAL_DIDSetPSA_raw8"
  [VHAL_DIDSetTNBCPSA_raw8] -> Bus Creator/41  "VHAL_DIDSetTNBCPSA_raw8"
  [VHAL_DIDSetTNECPSA_raw8] -> Bus Creator/42  "VHAL_DIDSetTNECPSA_raw8"
  [VHAL_DIDSetTEBPSA_raw8] -> Bus Creator/43  "VHAL_DIDSetTEBPSA_raw8"
  [VHAL_DIDSetTGEOVC_raw8] -> Bus Creator/44  "VHAL_DIDSetTGEOVC_raw8"
  [VHAL_DIDSetGECHGOVCDC_raw8] -> Bus Creator/45  "VHAL_DIDSetGECHGOVCDC_raw8"
  [VHAL_DIDSetGECHGOVCAC_raw8] -> Bus Creator/46  "VHAL_DIDSetGECHGOVCAC_raw8"
  [VHAL_DIDSetRESSV2XENNONPSA_raw8] -> Bus Creator/47  "VHAL_DIDSetRESSV2XENNONPSA_raw8"
  [VHAL_DIDSetPKE_raw8] -> Bus Creator/48  "VHAL_DIDSetPKE_raw8"
  [VHAL_DIDSetCDEODT_raw8] -> Bus Creator/49  "VHAL_DIDSetCDEODT_raw8"
  [VHAL_DIDSetAvgBattTempPSA_raw8] -> Bus Creator/50  "VHAL_DIDSetAvgBattTempPSA_raw8"
  [VHAL_DIDSetAvgBattTempOVC_raw8] -> Bus Creator/51  "VHAL_DIDSetAvgBattTempOVC_raw8"
  [VHAL_DIDSetAvgBattTempOFF_raw8] -> Bus Creator/52  "VHAL_DIDSetAvgBattTempOFF_raw8"
  [VHAL_DIDSetQTYPSATRIPS_raw8] -> Bus Creator/53  "VHAL_DIDSetQTYPSATRIPS_raw8"
  [VHAL_DIDSetRESSCNTDODRNGR_raw8] -> Bus Creator/54  "VHAL_DIDSetRESSCNTDODRNGR_raw8"
  [VHAL_DIDSetRESSCNTDODRNGL_raw8] -> Bus Creator/55  "VHAL_DIDSetRESSCNTDODRNGL_raw8"
  [VHAL_DIDSetETMATOE_raw8] -> Bus Creator/56  "VHAL_DIDSetETMATOE_raw8"
  [VHAL_DIDSetETMBTOE_raw8] -> Bus Creator/57  "VHAL_DIDSetETMBTOE_raw8"
  [VHAL_DIDSetRESSTIMESOCPSARNGR_raw8] -> Bus Creator/58  "VHAL_DIDSetRESSTIMESOCPSARNGR_raw8"
  [VHAL_DIDSetRESSTIMESOCPSARNGL_raw8] -> Bus Creator/59  "VHAL_DIDSetRESSTIMESOCPSARNGL_raw8"
  [VHAL_DIDSetRESSTIMESOCCHGRNGR_raw8] -> Bus Creator/60  "VHAL_DIDSetRESSTIMESOCCHGRNGR_raw8"
  [VHAL_DIDSetRESSTIMESOCCHGRNGL_raw8] -> Bus Creator/61  "VHAL_DIDSetRESSTIMESOCCHGRNGL_raw8"
  [VHAL_DIDSetRESSTIMESOCOFFRNGL_raw8] -> Bus Creator/63  "VHAL_DIDSetRESSTIMESOCOFFRNGL_raw8"
  [VHAL_DIDSetRESSTIMESOCOFFRNGR_raw8] -> Bus Creator/62  "VHAL_DIDSetRESSTIMESOCOFFRNGR_raw8"
  convert_in/1 -> uint32Touint8Array4/1(In1)
  [VOUTP_ODOMETER_km] -> convert_in/1
  [VOUTP_CDEODTR_km] -> convert_in12/1
  [VOUTP_CDEODTL_km] -> convert_in13/1
  [VOUTP_APPE_pct] -> convert_in28/1
  convert_in28/1 -> Data Type Conversion29/1
  convert_in29/1 -> Data Type Conversion27/1
  [VOUTP_APPD_pct] -> convert_in29/1
  [BOUTP_outputs] -> bus_selector/1
  BOUTP_outputs/1 -> [BOUTP_outputs]
  [BOUTP_outputs] -> Bus Selector/1
  [VHAL_DIDSetReadKeyIndexDataIdentifier_raw8] -> Bus Creator/64  "VHAL_DIDSetReadKeyIndexDataIdentifier_raw8"
  [VHAL_DIDSetDKCStatus_raw8] -> Bus Creator/65  "VHAL_DIDSetDKCSta_raw8"
  [VHAL_DIDSetBLEStatus_raw8] -> Bus Creator/66  "VHAL_DIDSetDKCBLESta_raw8"
  [VHAL_DIDSetUWBanchorStatus_raw8] -> Bus Creator/67  "VHAL_DIDSetUWBAnchorSta_raw8"
  [VHAL_DIDSetLIDAanchorStatus_raw8] -> Bus Creator/68  "VHAL_DIDSetLIDAAnchorSta_raw8"
  [VHAL_DIDSetDoorNFCanchorStatus_raw8] -> Bus Creator/69  "VHAL_DIDSetDoorNFCAnchorSta_raw8"
  [VHAL_DIDSetUIDStatus_raw8] -> Bus Creator/70  "VHAL_DIDSetUIDSta_raw8"
  [VHAL_DIDSetFDDKCCoordinateXY_raw8] -> Bus Creator/71  "VHAL_DIDSetFDDKCCoordXY_raw8"
  bus_selector/1 -> [DKCCurrentCarKeytype]  "<VOUTP_KeyModeSta_enum>"
  bus_selector/2 -> [DKCCurrentKeyfobposition]  "<VOUTP_UWBDetArea_enum>"
  bus_selector/3 -> [DKCBLERSSI]  "<VOUTP_BLERSSI_enum>"
  bus_selector/4 -> [DKCDKCUWBOnOffSta]  "<VOUTP_UWBOnOff_flg>"
  bus_selector/5 -> [DKCDKCUWB1InvalidSta]  "<VOUTP_UWB1Invalid_flg>"
  bus_selector/6 -> [DKCDKCUWB2InvalidSta]  "<VOUTP_UWB2Invalid_flg>"
  bus_selector/7 -> [DKCDKCUWB3InvalidSta]  "<VOUTP_UWB3Invalid_flg>"
  bus_selector/8 -> [DKCDKCUWB4InvalidSta]  "<VOUTP_UWB4Invalid_flg>"
  bus_selector/9 -> [DKCDKCUWB5InvalidSta]  "<VOUTP_UWB0Invalid_flg>"
  bus_selector/10 -> [DKCDKCUWB1FPPSta]  "<VOUTP_UWB1FPP_enum>"
  bus_selector/11 -> [DKCDKCUWB2FPPSta]  "<VOUTP_UWB2FPP_enum>"
  bus_selector/12 -> [DKCDKCUWB3FPPSta]  "<VOUTP_UWB3FPP_enum>"
  bus_selector/13 -> [DKCDKCUWB4FPPSta]  "<VOUTP_UWB4FPP_enum>"
  bus_selector/14 -> [DKCDKCUWB5FPPSta]  "<VOUTP_UWB0FPP_enum>"
  bus_selector/15 -> [DKCDKCUWB1DistanceSta]  "<VOUTP_UWB1Distance_enum>"
  bus_selector/16 -> [DKCDKCUWB2DistanceSta]  "<VOUTP_UWB2Distance_enum>"
  bus_selector/17 -> [DKCDKCUWB3DistanceSta]  "<VOUTP_UWB3Distance_enum>"
  bus_selector/18 -> [DKCDKCUWB4DistanceSta]  "<VOUTP_UWB4Distance_enum>"
  bus_selector/19 -> [DKCDKCUWB5DistanceSta]  "<VOUTP_UWB0Distance_enum>"
  bus_selector/20 -> [DKCUIDcurrentvoltage]  "<VOUTP_UIDBatVolt_enum>"
  bus_selector/21 -> [DKCFDCDKCCoordinateXSta]  "<VOUTP_CoordinateX_enum>"
  bus_selector/22 -> [DKCFDCDKCCoordinateYSta]  "<VOUTP_CoordinateY_enum>"
  [Byte_5_DKCUWB3FPPSta] -> Data Type Conversion108/1
  [Byte_10_DKCUWB3DistanceSta] -> Data Type Conversion114/1
  BitwiseOR66/1 -> [UWBanchorStatus10]
  Data Type Conversion135/1 -> BitwiseOR86/1
  Data Type Conversion107/1 -> BitwiseOR61/1
  Data Type Conversion116/1 -> BitwiseOR69/1
  [Byte_0_DKCUWBOnOffSta] -> Data Type Conversion99/1
  Data Type Conversion136/1 -> BitwiseOR87/1
  Mux32/1 -> [VHAL_DIDSetBLEStatus_raw8]
  BitwiseOR53/1 -> [DKCStatus1]
  Data Type Conversion95/1 -> BitwiseOR53/2
  Data Type Conversion94/1 -> BitwiseOR53/1
  [Byte_0_FDCDKCCoordinateXSta] -> Data Type Conversion141/1
  BitwiseOR57/1 -> [UWBanchorStatus1]
  [Byte_3_DKCUWB1FPPSta] -> Data Type Conversion106/1
  [Byte_4_DKCUWB2FPPSta] -> Data Type Conversion107/1
  BitwiseOR86/1 -> [UIDStatus3]
  [UWBanchorStatus21] -> Mux33/21
  Mux34/1 -> [VHAL_DIDSetLIDAanchorStatus_raw8]
  [LIDAanchorStatus1] -> Mux34/1
  [BLEStatus1] -> Mux32/1
  Data Type Conversion105/1 -> BitwiseOR59/1
  Data Type Conversion109/1 -> BitwiseOR63/1
  BitwiseOR58/1 -> [UWBanchorStatus2]
  Mux36/1 -> [VHAL_DIDSetUIDStatus_raw8]
  [UIDStatus8] -> Mux36/8
  [UIDStatus7] -> Mux36/7
  [FDDKCCoordinateXY1] -> Mux37/1
  BitwiseOR59/1 -> [UWBanchorStatus3]
  [Byte_21_UIDcurrentvoltage] -> Data Type Conversion136/1
  Data Type Conversion142/1 -> BitwiseOR93/1
  [UWBanchorStatus1] -> Mux33/1
  [DoorNFCanchorStatus3] -> Mux35/3
  Data Type Conversion113/1 -> BitwiseOR66/1
  [Byte_11_DKCUWB4DistanceSta] -> Data Type Conversion115/1
  [Byte_8_DKCUWB1DistanceSta] -> Data Type Conversion111/1
  BitwiseOR62/1 -> [UWBanchorStatus6]
  Data Type Conversion108/1 -> BitwiseOR62/1
  [Byte_12_DKCUWB5DistanceSta] -> Data Type Conversion116/1
  Mux31/1 -> [VHAL_DIDSetDKCStatus_raw8]
  [Byte_0_CurrentKeyfobposition] -> Data Type Conversion95/1
  [Byte_0_CurrentCarKeytype] -> Data Type Conversion94/1
  Data Type Conversion141/1 -> BitwiseOR92/1
  [DKCStatus1] -> Mux31/1
  [UWBanchorStatus6] -> Mux33/6
  [UWBanchorStatus15] -> Mux33/15
  [UWBanchorStatus13] -> Mux33/13
  [UWBanchorStatus3] -> Mux33/3
  [UWBanchorStatus2] -> Mux33/2
  [UWBanchorStatus8] -> Mux33/8
  [Byte_1_DKCUWB4InvalidSta] -> Data Type Conversion104/1
  [UWBanchorStatus7] -> Mux33/7
  [UWBanchorStatus5] -> Mux33/5
  [UWBanchorStatus17] -> Mux33/17
  [Byte_7_DKCUWB5FPPSta] -> Data Type Conversion110/1
  BitwiseOR92/1 -> [FDDKCCoordinateXY1]
  [Byte_2_FDCDKCCoordinateYSta] -> Data Type Conversion144/1
  BitwiseOR93/1 -> [FDDKCCoordinateXY2]
  [Byte_1_FDCDKCCoordinateYSta] -> Data Type Conversion143/1
  Data Type Conversion143/1 -> BitwiseOR93/2
  [FDDKCCoordinateXY2] -> Mux37/2
  [UWBanchorStatus18] -> Mux33/18
  [UIDStatus2] -> Mux36/2
  Data Type Conversion144/1 -> BitwiseOR94/1
  [FDDKCCoordinateXY3] -> Mux37/3
  Data Type Conversion111/1 -> BitwiseOR65/1
  BitwiseOR87/1 -> [UIDStatus4]
  BitwiseOR68/1 -> [UWBanchorStatus12]
  BitwiseOR69/1 -> [UWBanchorStatus13]
  BitwiseOR67/1 -> [UWBanchorStatus11]
  BitwiseOR65/1 -> [UWBanchorStatus9]
  Data Type Conversion114/1 -> BitwiseOR67/1
  [UWBanchorStatus20] -> Mux33/20
  [Byte_1_DKCUWB2InvalidSta] -> Data Type Conversion102/1
  Data Type Conversion104/1 -> BitwiseOR58/4
  Data Type Conversion115/1 -> BitwiseOR68/1
  [UIDStatus6] -> Mux36/6
  [DoorNFCanchorStatus1] -> Mux35/1
  [UWBanchorStatus10] -> Mux33/10
  [UWBanchorStatus16] -> Mux33/16
  [UWBanchorStatus14] -> Mux33/14
  [UWBanchorStatus19] -> Mux33/19
  Data Type Conversion99/1 -> BitwiseOR57/1
  Data Type Conversion110/1 -> BitwiseOR64/1
  [Byte_1_DKCUWB1InvalidSta] -> Data Type Conversion100/1
  [Byte_1_DKCUWB3InvalidSta] -> Data Type Conversion103/1
  [Byte_2_DKCUWB5InvalidSta] -> Data Type Conversion105/1
  [Byte_1_FDCDKCCoordinateXSta] -> Data Type Conversion142/1
  BitwiseOR61/1 -> [UWBanchorStatus5]
  [UWBanchorStatus11] -> Mux33/11
  [UIDStatus5] -> Mux36/5
  [UWBanchorStatus9] -> Mux33/9
  [Byte_20_UIDcurrentvoltage] -> Data Type Conversion135/1
  [DoorNFCanchorStatus2] -> Mux35/2
  BitwiseOR63/1 -> [UWBanchorStatus7]
  BitwiseOR56/1 -> [BLEStatus2]
  BitwiseOR64/1 -> [UWBanchorStatus8]
  [UWBanchorStatus12] -> Mux33/12
  [UIDStatus4] -> Mux36/4
  Mux37/1 -> [VHAL_DIDSetFDDKCCoordinateXY_raw8]
  BitwiseOR94/1 -> [FDDKCCoordinateXY3]
  Data Type Conversion98/1 -> BitwiseOR56/1
  Data Type Conversion103/1 -> BitwiseOR58/3
  [LIDAanchorStatus2] -> Mux34/2
  [DKCStatus2] -> Mux31/2
  [Byte_9_DKCUWB2DistanceSta] -> Data Type Conversion113/1
  Mux33/1 -> [VHAL_DIDSetUWBanchorStatus_raw8]
  Data Type Conversion106/1 -> BitwiseOR60/1
  [Byte_6_DKCUWB4FPPSta] -> Data Type Conversion109/1
  Data Type Conversion102/1 -> BitwiseOR58/2
  BitwiseOR60/1 -> [UWBanchorStatus4]
  [BLEStatus2] -> Mux32/2
  [UIDStatus3] -> Mux36/3
  [UIDStatus1] -> Mux36/1
  [UWBanchorStatus4] -> Mux33/4
  [LIDAanchorStatus3] -> Mux34/3
  [Byte_1_BLERSSI] -> Data Type Conversion98/1
  Data Type Conversion100/1 -> BitwiseOR58/1
  Constant3/1 -> [UWBanchorStatus14]
  Constant4/1 -> [UWBanchorStatus15]
  Constant5/1 -> [UWBanchorStatus16]
  Constant6/1 -> [UWBanchorStatus17]
  Constant7/1 -> [UWBanchorStatus18]
  Constant8/1 -> [UWBanchorStatus19]
  Constant9/1 -> [UWBanchorStatus20]
  Constant10/1 -> [UWBanchorStatus21]
  Constant11/1 -> [LIDAanchorStatus3]
  Constant13/1 -> [LIDAanchorStatus2]
  Constant12/1 -> [LIDAanchorStatus1]
  Constant15/1 -> [DoorNFCanchorStatus1]
  Constant16/1 -> [DoorNFCanchorStatus2]
  Constant14/1 -> Goto191/1
  Constant17/1 -> [UIDStatus2]
  Constant18/1 -> [UIDStatus1]
  Constant23/1 -> [UIDStatus7]
  Constant22/1 -> [UIDStatus8]
  Constant19/1 -> [UIDStatus6]
  Constant21/1 -> [UIDStatus5]
  Mux35/1 -> [VHAL_DIDSetDoorNFCanchorStatus_raw8]
  convert_out61/1 -> UnitConverter60/1
  [DKCBLERSSI] -> convert_out61/1
  [DKCUIDcurrentvoltage] -> convert_out97/1
  convert_out97/1 -> UnitConverter93/1
  UnitConverter97/1 -> RightShift8/1, RightShift9/1
  convert_out101/1 -> UnitConverter97/1
  RightShift6/1 -> BitwiseAND69/1
  UnitConverter64/1 -> LeftShift48/1
  BitwiseAND47/1 -> [Byte_1_DKCUWB2InvalidSta]
  LeftShift47/1 -> BitwiseAND47/1
  convert_out100/1 -> UnitConverter96/1
  BitwiseAND45/1 -> [Byte_0_DKCUWBOnOffSta]
  LeftShift45/1 -> BitwiseAND45/1
  LeftShift51/1 -> BitwiseAND51/1
  UnitConverter67/1 -> LeftShift51/1
  convert_out66/1 -> UnitConverter65/1
  [DKCDKCUWB4InvalidSta] -> convert_out66/1
  BitwiseAND46/1 -> [Byte_1_DKCUWB1InvalidSta]
  BitwiseAND51/1 -> [Byte_3_DKCUWB1FPPSta]
  LeftShift46/1 -> BitwiseAND46/1
  UnitConverter62/1 -> LeftShift46/1
  UnitConverter74/1 -> LeftShift58/1
  BitwiseAND59/1 -> [Byte_11_DKCUWB4DistanceSta]
  BitwiseAND57/1 -> [Byte_9_DKCUWB2DistanceSta]
  convert_out74/1 -> UnitConverter72/1
  [DKCDKCUWB1DistanceSta] -> convert_out74/1
  BitwiseAND58/1 -> [Byte_10_DKCUWB3DistanceSta]
  [DKCFDCDKCCoordinateXSta] -> convert_out100/1
  BitwiseAND50/1 -> [Byte_2_DKCUWB5InvalidSta]
  UnitConverter75/1 -> LeftShift59/1
  UnitConverter66/1 -> LeftShift50/1
  BitwiseAND56/1 -> [Byte_8_DKCUWB1DistanceSta]
  BitwiseAND49/1 -> [Byte_1_DKCUWB4InvalidSta]
  LeftShift49/1 -> BitwiseAND49/1
  UnitConverter65/1 -> LeftShift49/1
  convert_out72/1 -> UnitConverter70/1
  [DKCDKCUWB4FPPSta] -> convert_out72/1
  [DKCDKCUWB3FPPSta] -> convert_out70/1
  convert_out65/1 -> UnitConverter64/1
  [DKCDKCUWB3InvalidSta] -> convert_out65/1
  LeftShift57/1 -> BitwiseAND57/1
  UnitConverter61/1 -> LeftShift45/1
  [DKCDKCUWBOnOffSta] -> convert_out62/1
  [DKCDKCUWB2InvalidSta] -> convert_out64/1
  [DKCDKCUWB1InvalidSta] -> convert_out63/1
  convert_out62/1 -> UnitConverter61/1
  LeftShift50/1 -> BitwiseAND50/1
  convert_out69/1 -> UnitConverter68/1
  UnitConverter93/1 -> RightShift/1, RightShift1/1
  BitwiseAND72/1 -> [Byte_2_FDCDKCCoordinateYSta]
  RightShift9/1 -> BitwiseAND72/1
  RightShift7/1 -> BitwiseAND70/1
  [DKCDKCUWB2FPPSta] -> convert_out69/1
  RightShift1/1 -> BitwiseAND64/1
  BitwiseAND63/1 -> [Byte_20_UIDcurrentvoltage]
  RightShift/1 -> BitwiseAND63/1
  convert_out78/1 -> UnitConverter76/1
  convert_out64/1 -> UnitConverter63/1
  [DKCDKCUWB5DistanceSta] -> convert_out78/1
  convert_out77/1 -> UnitConverter75/1
  [DKCDKCUWB4DistanceSta] -> convert_out77/1
  BitwiseAND64/1 -> [Byte_21_UIDcurrentvoltage]
  BitwiseAND60/1 -> [Byte_12_DKCUWB5DistanceSta]
  LeftShift60/1 -> BitwiseAND60/1
  UnitConverter63/1 -> LeftShift47/1
  BitwiseAND70/1 -> [Byte_1_FDCDKCCoordinateXSta]
  LeftShift48/1 -> BitwiseAND48/1
  convert_out70/1 -> UnitConverter69/1
  convert_out68/1 -> UnitConverter67/1
  convert_out73/1 -> UnitConverter71/1
  [DKCDKCUWB5FPPSta] -> convert_out73/1
  [DKCDKCUWB1FPPSta] -> convert_out68/1
  convert_out67/1 -> UnitConverter66/1
  convert_out75/1 -> UnitConverter73/1
  [DKCDKCUWB2DistanceSta] -> convert_out75/1
  BitwiseAND53/1 -> [Byte_5_DKCUWB3FPPSta]
  LeftShift53/1 -> BitwiseAND53/1
  LeftShift55/1 -> BitwiseAND55/1
  UnitConverter71/1 -> LeftShift55/1
  LeftShift52/1 -> BitwiseAND52/1
  UnitConverter68/1 -> LeftShift52/1
  BitwiseAND54/1 -> [Byte_6_DKCUWB4FPPSta]
  LeftShift54/1 -> BitwiseAND54/1
  [DKCDKCUWB3DistanceSta] -> convert_out76/1
  convert_out63/1 -> UnitConverter62/1
  LeftShift59/1 -> BitwiseAND59/1
  UnitConverter69/1 -> LeftShift53/1
  LeftShift40/1 -> BitwiseAND40/1
  LeftShift58/1 -> BitwiseAND58/1
  BitwiseAND40/1 -> [Byte_0_CurrentCarKeytype]
  UnitConverter73/1 -> LeftShift57/1
  UnitConverter56/1 -> LeftShift40/1
  BitwiseAND41/1 -> [Byte_0_CurrentKeyfobposition]
  UnitConverter57/1 -> LeftShift41/1
  UnitConverter76/1 -> LeftShift60/1
  [DKCFDCDKCCoordinateYSta] -> convert_out101/1
  UnitConverter96/1 -> RightShift6/1, RightShift7/1
  RightShift8/1 -> BitwiseAND71/1
  UnitConverter72/1 -> LeftShift56/1
  BitwiseAND71/1 -> [Byte_1_FDCDKCCoordinateYSta]
  BitwiseAND44/1 -> [Byte_1_BLERSSI]
  BitwiseAND69/1 -> [Byte_0_FDCDKCCoordinateXSta]
  UnitConverter60/1 -> LeftShift44/1
  [DKCCurrentKeyfobposition] -> convert_out57/1
  UnitConverter70/1 -> LeftShift54/1
  [DKCCurrentCarKeytype] -> convert_out56/1
  LeftShift44/1 -> BitwiseAND44/1
  convert_out56/1 -> UnitConverter56/1
  BitwiseAND55/1 -> [Byte_7_DKCUWB5FPPSta]
  LeftShift56/1 -> BitwiseAND56/1
  BitwiseAND52/1 -> [Byte_4_DKCUWB2FPPSta]
  BitwiseAND48/1 -> [Byte_1_DKCUWB3InvalidSta]
  LeftShift41/1 -> BitwiseAND41/1
  [DKCDKCUWB5InvalidSta] -> convert_out67/1
  convert_out76/1 -> UnitConverter74/1
  convert_out57/1 -> UnitConverter57/1
